simulink model "lab2_2"  (R2021a)
settings: Solver=ode23t  StartTime=0.0  StopTime=0.1  MaxStep=1e-5  RelTol=1e-3
libraries: spsRMSLib x8, spsFourierLib x4, spsVoltageMeasurementLib x3, spsCurrentMeasurementLib x2, spsMeanLib x2, spsSeriesRLCBranchLib x2, spsThyristorLib x2, spsACVoltageSourceLib x1, spsControlledCurrentSourceLib x1, simulink x1, spsMosfetLib x1, spsPowerLib x1
settings Model: Creator=up1072827  LastModifiedBy=Rigas
settings DataIOCC: ReturnWorkspaceOutputs=off

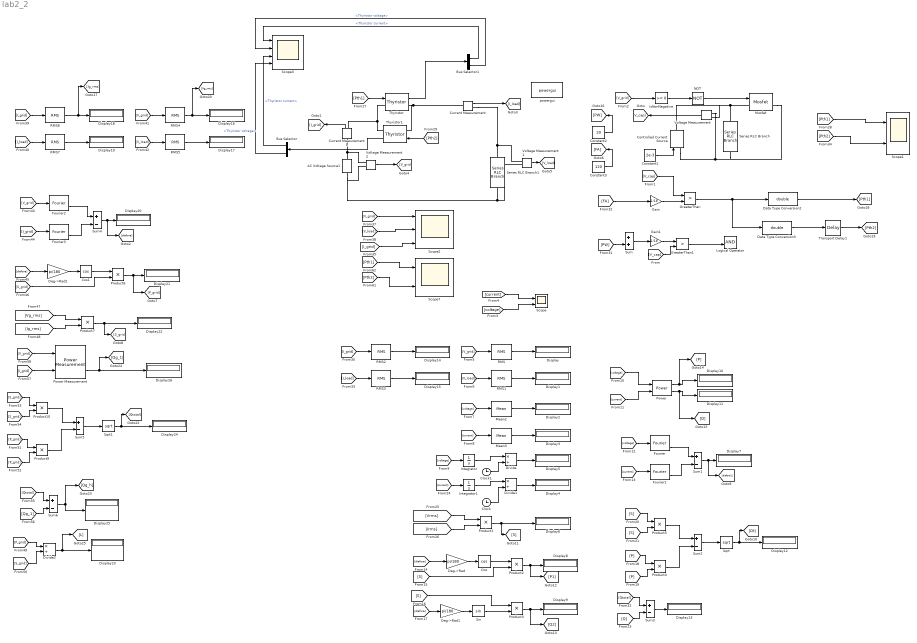
== system lab2_2 ==
  AC Voltage Source1 : spsACVoltageSourceLib/AC Voltage Source  Amplitude=230*sqrt(2)  Phase=0  Frequency=50  SampleTime=0  Measurements=None  BusType=swing  Pref=10e3  Qref=0  Qmin=-inf  Qmax=+inf
  Bus Selector : BusSelector  OutputSignals=Thyristor current,Thyristor voltage
  Bus Selector1 : BusSelector  OutputSignals=Thyristor current,Thyristor voltage
  Clock : Clock
  Clock1 : Clock
  Constant1 : Constant  Value=2e-3
  Constant2 : Constant  Value=20
  Constant3 : Constant  Value=120
  Controlled Current Source : spsControlledCurrentSourceLib/Controlled Current Source  Initialize=on  Source_Type=AC  Amplitude=0  Phase=0  Frequency=0  Measurements=None
  Cos : Trigonometry  Operator=cos
  Cos1 : Trigonometry  Operator=cos
  Current Measurement : spsCurrentMeasurementLib/Current Measurement  PhasorSimulation=off  OutputType=Complex  PSBequivalent=0
  Current Measurement1 : spsCurrentMeasurementLib/Current Measurement  PhasorSimulation=off  OutputType=Complex  PSBequivalent=0
  Data Type Conversion2 : DataTypeConversion  OutDataTypeStr=double
  Data Type Conversion3 : DataTypeConversion  OutDataTypeStr=double
  Deg->Rad : Gain  Gain=pi/180  SaturateOnIntegerOverflow=on  OutDataTypeStr=Inherit: Same as input  ParamDataTypeStr=Inherit: Same as input
  Deg->Rad1 : Gain  Gain=pi/180  SaturateOnIntegerOverflow=on  OutDataTypeStr=Inherit: Same as input  ParamDataTypeStr=Inherit: Same as input
  Deg->Rad2 : Gain  Gain=pi/180  SaturateOnIntegerOverflow=on  OutDataTypeStr=Inherit: Same as input  ParamDataTypeStr=Inherit: Same as input
  Display{,1..26} (27 alike) : Display
  Divide : Product  Inputs=*/
  Divide1 : Product  Inputs=*/
  Divide2 : Product  Inputs=*/
  Fourier{,1..3} (4 alike) : spsFourierLib/Fourier  Freq=50  n=1  InInit=[0, 0]  Ts=0
      settings: SourceProductBaseCode=PS
  Gain : Gain  Gain=1/18
  Gain1 : Gain  Gain=1/18
  GreaterThan : RelationalOperator  Operator=>  OutDataTypeStr=boolean  RndMeth=Simplest
  GreaterThan1 : RelationalOperator  Operator=>  OutDataTypeStr=boolean  RndMeth=Simplest
  Integrator : Integrator
  Integrator1 : Integrator
  IsNonNegative : simulink/Logic and Bit Operations/Compare To Zero  relop=>=  OutDataTypeStr=boolean
  Logical Operator : Logic  AllPortsSameDT=off  OutDataTypeStr=boolean
  Mean2 : spsMeanLib/Mean  Freq=50  Vinit=0  Ts=0
  Mean3 : spsMeanLib/Mean  Freq=50  Vinit=0  Ts=0
  Mosfet : spsMosfetLib/Mosfet  Ron=0.1  Lon=0  Rd=0.01  Vfd=0  IC=0  Rs=1e5  Cs=inf  Measurements=on
  NOT : Logic  Operator=NOT  IconShape=distinctive  AllPortsSameDT=off  OutDataTypeStr=boolean
  Power : spsPowerLib/Power  Freq=50  Vinit=[1, 0]  Iinit=[1, 0]  Ts=0
      settings: SourceProductBaseCode=PS
  Power Measurement : eePowerMeasurement/Power Measurement  LabelModeActiveChoice=Continuous  F=50  K=[1]  Ts=0
      settings: SourceProductBaseCode=PS
  Product{1..7,9..10} (9 alike) : Product
  RMS{,1..7} (8 alike) : spsRMSLib/RMS  TrueRMS=on  Freq=50  RMSInit=120  Ts=0
  Scope : Scope  NumInputPorts=2
  Scope1 : Scope  NumInputPorts=2
  Scope2 : Scope  NumInputPorts=3
  Scope3 : Scope  NumInputPorts=4
  Scope7 : Scope  NumInputPorts=2
  Series RLC Branch : spsSeriesRLCBranchLib/Series RLC Branch  LConnTagsString=__new0  RConnTagsString=__new0  BranchType=RC  Resistance=1e-3  Inductance=2e-6  SetiL0=off  InitialCurrent=0  Capacitance=1.95e-6  Setx0=off  InitialVoltage=0  Measurements=None
  Series RLC Branch1 : spsSeriesRLCBranchLib/Series RLC Branch  LConnTagsString=__new0  RConnTagsString=__new0  BranchType=RL  Resistance=50  Inductance=275.66e-3  SetiL0=off  InitialCurrent=0  Capacitance=1e-6  Setx0=off  InitialVoltage=0  Measurements=None
  Sin : Trigonometry
  Sqrt : Sqrt  SaturateOnIntegerOverflow=on
  Sqrt1 : Sqrt  SaturateOnIntegerOverflow=on
  Sum : Sum  InputSameDT=on  SaturateOnIntegerOverflow=on  OutDataTypeStr=Inherit: Same as first input
  Sum{1..6} (6 alike) : Sum  Inputs=+-  InputSameDT=on  SaturateOnIntegerOverflow=on  OutDataTypeStr=Inherit: Same as first input
  Thyristor : spsThyristorLib/Thyristor  Ron=0.001  Lon=0  Vf=0.8  IC=0  Rs=500  Cs=250e-9  Measurements=on
  Thyristor1 : spsThyristorLib/Thyristor  Ron=0.001  Lon=0  Vf=0.8  IC=0  Rs=500  Cs=250e-9  Measurements=on
  Transport Delay1 : TransportDelay  DelayTime=0.01
  Voltage Measurement : spsVoltageMeasurementLib/Voltage Measurement  PhasorSimulation=off  OutputType=Complex  PSBequivalent=0
  Voltage Measurement1 : spsVoltageMeasurementLib/Voltage Measurement  PhasorSimulation=off  OutputType=Complex  PSBequivalent=0
  Voltage Measurement2 : spsVoltageMeasurementLib/Voltage Measurement  PhasorSimulation=off  OutputType=Complex  PSBequivalent=0
  powergui : spspowerguiLib/powergui  Priority=1  SimulationMode=Continuous  SampleTime=1e-5  frequency=60  Iterations=50  frequencyindice=50  Pbase=100e6  ErrMax=1e-4  UnitsV=kV  UnitsW=MW  buscounter=0  FunctionMessages=off  echomessages=off  EnableUseOfTLC=off  CurrentSourceSwitches=off  DisableSnubberDevices=on  DisableRonSwitches=on  DisableVfSwitches=on  DisplayEquations=off  AutomaticDiscreteSolvers=off  SolverType=Tustin/Backward Euler (TBE)  Interpol=off  ExternalGateDelay=off  methode=off  Ts=100  x0status=blocks  SPID=on  SwTol=0  HookPort=off  NonlinearTolerance=1e-4  nMaxIteration=100  ContinueOnMaxIteration=off  RestoreLinks=warning  ResistiveCurrentMeasurement=off  Frange=[0:2:500]  Ylog=off  Xlog=on  ShowGrid=off  save=off  variable=ZData  structure=0  ZoomFFT=off  StartTime=0.0  cycles=1  DisplayStyle=1  fundamental=60  FreqAxis=off  MaxFrequency=1000  frequencyindicesteady=1  RmsSteady=1  display=off
  wires:
  IsNonNegative/1 -> NOT/1
  NOT/1 -> Mosfet/1
  Gain/1 -> GreaterThan/2
  Gain1/1 -> GreaterThan1/1
  GreaterThan1/1 -> Logical Operator/2
  [V_cap] -> GreaterThan1/2
  Sum/1 -> Gain1/1
  [V_cap] -> GreaterThan/1
  [PW] -> Sum/2
  Constant1/1 -> Controlled Current Source/1
  Current Measurement/1 -> [I_load]
  Voltage Measurement2/1 -> [V_grid]
  Voltage Measurement1/1 -> [V_load]
  [V_grid] -> IsNonNegative/1
  Sum3/1 -> Display13/1
  Product3/1 -> [Q2], Display9/1
  [current] -> Mean3/1
  [S] -> Product5/2
  Mean3/1 -> Display3/1
  Sin/1 -> Product3/2
  [Q] -> Sum3/2
  Product1/1 -> [S], Display6/1
  Fourier1/2 -> Sum1/2
  [voltage] -> Power/1
  Sqrt/1 -> [Qt], Display12/1
  [voltage] -> Scope/2
  Product4/1 -> Sum2/2
  [S] -> Product5/1
  RMS/1 -> Display/1
  [P] -> Product4/1
  Power/1 -> [P], Display10/1
  Product2/1 -> [P1], Display8/1
  Deg->Rad1/1 -> Sin/1
  Sum2/1 -> Sqrt/1
  [diafora] -> Deg->Rad1/1
  Cos/1 -> Product2/1
  [S] -> Product3/1
  [S] -> Product2/2
  [P] -> Product4/2
  Integrator1/1 -> Divide1/1
  [diafora] -> Deg->Rad/1
  [current] -> Scope/1
  Clock1/1 -> Divide/2
  [current] -> Fourier1/1
  [Irms] -> Product1/2
  Power/2 -> [Q], Display11/1
  Product5/1 -> Sum2/1
  Fourier/2 -> Sum1/1
  Deg->Rad/1 -> Cos/1
  [current] -> Power/2
  Sum1/1 -> [diafora1], Display7/1
  [voltage] -> Fourier/1
  [Vrms] -> Product1/1
  Divide/1 -> Display5/1
  [voltage] -> Mean2/1
  RMS1/1 -> Display1/1
  Clock/1 -> Divide1/2
  [Qtotal] -> Sum3/1
  [V_load] -> RMS1/1
  Integrator/1 -> Divide/1
  [V_grid] -> RMS/1
  Mean2/1 -> Display2/1
  [current] -> Integrator1/1
  Divide1/1 -> Display4/1
  [voltage] -> Integrator/1
  [Pth1] -> Scope1/1
  Voltage Measurement/1 -> [V_cap]
  Constant2/1 -> [PW]
  Constant3/1 -> [FA]
  [FA] -> Gain/1
  Data Type Conversion2/1 -> [Pth1]
  Data Type Conversion3/1 -> Transport Delay1/1
  Transport Delay1/1 -> [Pth2]
  [Pth2] -> Scope1/2
  [Pth1] -> Thyristor/1
  [Pth2] -> Thyristor1/1
  Current Measurement1/1 -> [I_grid]
  [I_grid] -> RMS2/1
  RMS2/1 -> Display14/1
  [I_load] -> RMS3/1
  RMS3/1 -> Display15/1
  GreaterThan/1 -> Data Type Conversion3/1, Data Type Conversion2/1
  [I_load] -> RMS7/1
  [V_grid] -> RMS4/1
  RMS4/1 -> [Vg_rms], Display16/1
  [V_load] -> RMS5/1
  [I_grid] -> RMS6/1
  RMS6/1 -> [Ig_rms], Display18/1
  RMS7/1 -> Display19/1
  RMS5/1 -> Display17/1
  Fourier3/2 -> Sum4/2
  Sum4/1 -> [diafora], Display20/1
  [V_grid] -> Fourier2/1
  Fourier2/2 -> Sum4/1
  [I_grid] -> Fourier3/1
  [diafora] -> Deg->Rad2/1
  Deg->Rad2/1 -> Cos1/1
  [S_grid] -> Product6/2
  Cos1/1 -> Product6/1
  Product6/1 -> [P_grid], Display21/1
  [Ig_rms] -> Product7/2
  [Vg_rms] -> Product7/1
  Product7/1 -> [S_grid], Display22/1
  Product10/1 -> Sum5/1
  Sum5/1 -> Sqrt1/1
  [P_grid] -> Product9/2
  [P_grid] -> Product9/1
  [S_grid] -> Product10/2
  Sqrt1/1 -> [Qtotal], Display24/1
  Product9/1 -> Sum5/2
  [S_grid] -> Product10/1
  [Qtotal] -> Sum6/1
  [Qg_1] -> Sum6/2
  Sum6/1 -> [Qg_h], Display25/1
  [V_grid] -> Power Measurement/1
  [I_grid] -> Power Measurement/2
  Power Measurement/2 -> Display26/1, [Qg_1]
  [P_grid] -> Divide2/1
  [S_grid] -> Divide2/2
  Divide2/1 -> [L], Display23/1
  Thyristor1/1 -> Bus Selector/1
  Thyristor/1 -> Bus Selector1/1
  Bus Selector/2 -> Scope3/4  "<Thyristor voltage>"
  Bus Selector/1 -> Scope3/3  "<Thyristor current>"
  Bus Selector1/1 -> Scope3/1  "<Thyristor current>"
  Bus Selector1/2 -> Scope3/2  "<Thyristor voltage>"
  [V_grid] -> Scope2/1
  [V_load] -> Scope2/2
  [I_grid] -> Scope2/3
  [Pth1] -> Scope7/1
  [Pth2] -> Scope7/2
  connections:
  Voltage Measurement/LConn1 -- Controlled Current Source/RConn1 -- Series RLC Branch/LConn1 -- Mosfet/LConn1
  Controlled Current Source/LConn1 -- Series RLC Branch/RConn1 -- Mosfet/RConn1 -- Voltage Measurement/LConn2
  Current Measurement/RConn1 -- Voltage Measurement1/LConn1 -- Series RLC Branch1/LConn1
  Voltage Measurement1/LConn2 -- Series RLC Branch1/RConn1 -- AC Voltage Source1/LConn1 -- Voltage Measurement2/LConn2
  Thyristor/RConn1 -- Thyristor1/LConn1 -- Current Measurement/LConn1
  AC Voltage Source1/RConn1 -- Current Measurement1/LConn1 -- Voltage Measurement2/LConn1
  Thyristor/LConn1 -- Current Measurement1/RConn1 -- Thyristor1/RConn1
